simulink model "FromWorkSpace_interp_extrap_struct"  (R2017b)
settings: Solver=FixedStepDiscrete  StartTime=0.0  StopTime=4  FixedStep=0.100000  RelTol=1e-3
model workspace (MAT data in the model file):
  Var = 0
  matrix_X.time = [1 2 3 4 5 6 7 8 9 10]
  matrix_X.signals.values = [3; 4; 5; 6; 7; 8; 9; 20; 32; 33]
  matrix_X.signals.dimensions = 1
settings Model: Creator=hbourbou  LastModifiedBy=hbourbou
settings DataIOCC: SaveFormat=StructureWithTime
settings OptimizationCC: LifeSpan=inf
settings DebuggingCC: SFExecutionAtInitializationDiag=none
settings HardwareCC: ProdBitPerSizeT=32  ProdBitPerPtrDiffT=32  ProdWordSize=32  ProdHWDeviceType=Specified
settings CodeAppCC: StateflowObjectComments=on

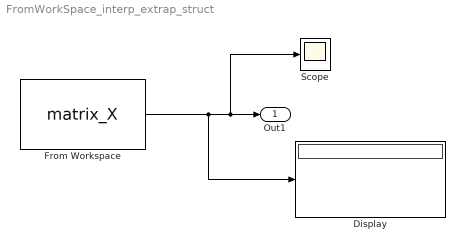
== system FromWorkSpace_interp_extrap_struct ==
  Display : Display
  From Workspace : FromWorkspace  VariableName=matrix_X  SampleTime=.1
  Scope : Scope
  Out1 : Outport
  wires:
  From Workspace/1 -> Display/1, Scope/1, Out1/1
